simulink model "p2"  (R2020b)
settings: Solver=VariableStepAuto  StartTime=0.0  StopTime=10  RelTol=1e-3
undefined symbols (not defined in the file): A, A1, B, B1, C, C1, K, K1, KDelay, L
settings Model: Creator=Julian  LastModifiedBy=Julian

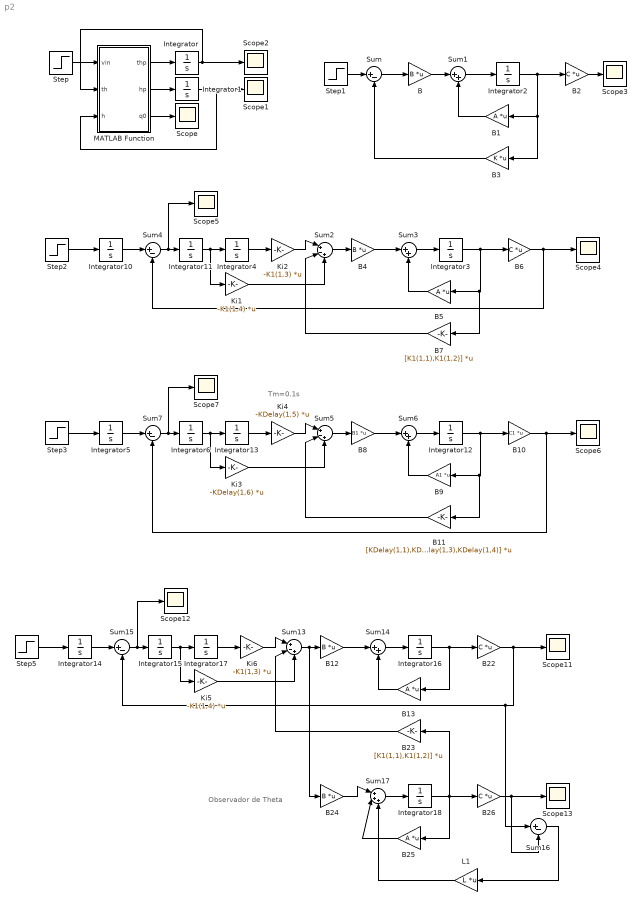
== system p2 ==
  note: Observador de Theta
  note: Tm=0.1s
  B{,4,12,24} (4 alike) : Gain  Gain=B  Multiplication=Matrix(K*u)
  B{1,5,13,25} (4 alike) : Gain  Gain=A  Multiplication=Matrix(K*u)
  B10 : Gain  Gain=C1  Multiplication=Matrix(K*u)
  B11 : Gain  Gain=[KDelay(1,1),KDelay(1,2),KDelay(1,3),KDelay(1,4)]  Multiplication=Matrix(K*u)
  B{2,6,22,26} (4 alike) : Gain  Gain=C  Multiplication=Matrix(K*u)
  B23 : Gain  Gain=[K1(1,1),K1(1,2)]  Multiplication=Matrix(K*u)
  B3 : Gain  Gain=K  Multiplication=Matrix(K*u)
  B7 : Gain  Gain=[K1(1,1),K1(1,2)]  Multiplication=Matrix(K*u)
  B8 : Gain  Gain=B1  Multiplication=Matrix(K*u)
  B9 : Gain  Gain=A1  Multiplication=Matrix(K*u)
  Integrator{,1..6,10..18} (16 alike) : Integrator
  Ki1 : Gain  Gain=-K1(1,4)  Multiplication=Matrix(K*u)
  Ki2 : Gain  Gain=-K1(1,3)  Multiplication=Matrix(K*u)
  Ki3 : Gain  Gain=-KDelay(1,6)  Multiplication=Matrix(K*u)
  Ki4 : Gain  Gain=-KDelay(1,5)  Multiplication=Matrix(K*u)
  Ki5 : Gain  Gain=-K1(1,4)  Multiplication=Matrix(K*u)
  Ki6 : Gain  Gain=-K1(1,3)  Multiplication=Matrix(K*u)
  L1 : Gain  Gain=L  Multiplication=Matrix(K*u)
  MATLAB Function : MATLAB Function  TreatAsAtomicUnit=on
  Scope{,1..7,11..13} (11 alike) : Scope
  Step{,1..2,5} (4 alike) : Step  Time=0  SampleTime=0
  Step3 : Step  Time=0.1  SampleTime=0
  Sum{,4,7,15..16} (5 alike) : Sum  Inputs=|+-
  Sum{1,3,6,14} (4 alike) : Sum  Inputs=|++
  Sum13 : Sum  Inputs=|+-+
  Sum17 : Sum  Inputs=|+++
  Sum2 : Sum  Inputs=|+-+
  Sum5 : Sum  Inputs=|+-+
  wires:
  MATLAB Function/1(thp) -> Integrator/1
  MATLAB Function/2(hp) -> Integrator1/1
  Integrator1/1 -> Scope1/1, MATLAB Function/3(h)
  Integrator/1 -> Scope2/1, MATLAB Function/2(th)
  Step/1 -> MATLAB Function/1(vin)
  MATLAB Function/3(q0) -> Scope/1
  Sum/1 -> B/1
  B/1 -> Sum1/1
  Sum1/1 -> Integrator2/1
  Integrator2/1 -> B2/1, B3/1, B1/1
  B1/1 -> Sum1/2
  B3/1 -> Sum/2
  Step1/1 -> Sum/1
  B2/1 -> Scope3/1
  B6/1 -> Sum4/2, Scope4/1
  B4/1 -> Sum3/1
  B7/1 -> Sum2/2
  Sum2/1 -> B4/1
  B5/1 -> Sum3/2
  Integrator3/1 -> B6/1, B7/1, B5/1
  Sum3/1 -> Integrator3/1
  Integrator4/1 -> Ki2/1
  Ki2/1 -> Sum2/1
  Sum4/1 -> Scope5/1, Integrator11/1
  Step2/1 -> Integrator10/1
  Integrator10/1 -> Sum4/1
  Integrator11/1 -> Ki1/1, Integrator4/1
  Ki1/1 -> Sum2/3
  Integrator6/1 -> Ki3/1, Integrator13/1
  B9/1 -> Sum6/2
  Integrator5/1 -> Sum7/1
  Ki3/1 -> Sum5/3
  Sum7/1 -> Scope7/1, Integrator6/1
  Integrator12/1 -> B10/1, B11/1, B9/1
  Step3/1 -> Integrator5/1
  Integrator13/1 -> Ki4/1
  B8/1 -> Sum6/1
  Sum6/1 -> Integrator12/1
  B11/1 -> Sum5/2
  Sum5/1 -> B8/1
  Ki4/1 -> Sum5/1
  B10/1 -> Scope6/1, Sum7/2
  B13/1 -> Sum14/2
  Ki5/1 -> Sum13/3
  Integrator14/1 -> Sum15/1
  Integrator15/1 -> Ki5/1, Integrator17/1
  Integrator17/1 -> Ki6/1
  Sum14/1 -> Integrator16/1
  Sum15/1 -> Scope12/1, Integrator15/1
  Integrator16/1 -> B22/1, B13/1
  B12/1 -> Sum14/1
  Step5/1 -> Integrator14/1
  Ki6/1 -> Sum13/1
  B23/1 -> Sum13/2
  Sum16/1 -> L1/1
  B26/1 -> Sum16/2, Scope13/1
  Integrator18/1 -> B23/1, B26/1, B25/1
  L1/1 -> Sum17/3
  Sum17/1 -> Integrator18/1
  B25/1 -> Sum17/2
  B22/1 -> Sum16/1, Sum15/2, Scope11/1
  Sum13/1 -> B24/1, B12/1
  B24/1 -> Sum17/1

== matlab function p2/MATLAB Function ==
  data: vin input; thp output; th input; h input; hp output; q0 output
function [thp,hp,q0] = fcn(vin,th,h)

ia=1;
kw=0.1;
C=1;
k=50;

thp=(1/kw)*(50*vin-10*ia);
hp=(1/C)*(80*th-k*sqrt(h));
q0=k*sqrt(h);
